simulink model "main_model"  (R2016a)
settings: Solver=VariableStepAuto  StartTime=0.0  StopTime=10.0  RelTol=1e-3
undefined symbols (not defined in the file): K, K_e, K_i
settings Model: Creator=manuel  LastModifiedBy=manuel

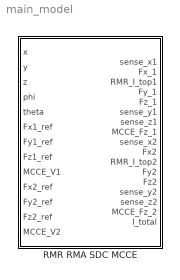
== system main_model ==
  RMR RMA SDC MCCE : Subsystem

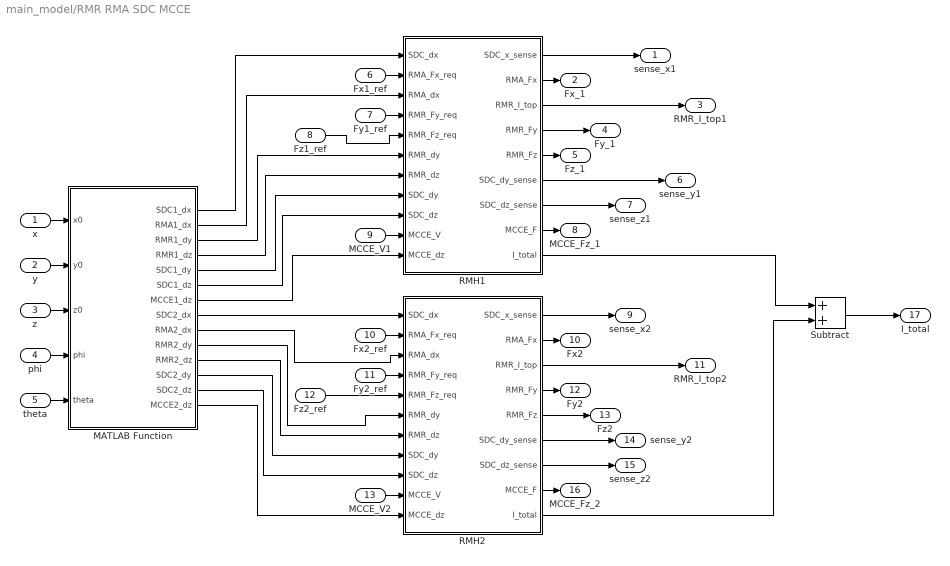
== system main_model/RMR RMA SDC MCCE ==
  x : Inport
  y : Inport  Port=2
  z : Inport  Port=3
  phi : Inport  Port=4
  theta : Inport  Port=5
  Fx1_ref : Inport  Port=6
  Fy1_ref : Inport  Port=7
  Fz1_ref : Inport  Port=8
  MCCE_V1 : Inport  Port=9
  Fx2_ref : Inport  Port=10
  Fy2_ref : Inport  Port=11
  Fz2_ref : Inport  Port=12
  MCCE_V2 : Inport  Port=13
  MATLAB Function : MATLAB Function  TreatAsAtomicUnit=on
  RMH1 : Subsystem
  RMH2 : Subsystem
  Subtract : Sum
  sense_x1 : Outport
  Fx_1 : Outport  Port=2
  RMR_I_top1 : Outport  Port=3
  Fy_1 : Outport  Port=4
  Fz_1 : Outport  Port=5
  sense_y1 : Outport  Port=6
  sense_z1 : Outport  Port=7
  MCCE_Fz_1 : Outport  Port=8
  sense_x2 : Outport  Port=9
  Fx2 : Outport  Port=10
  RMR_I_top2 : Outport  Port=11
  Fy2 : Outport  Port=12
  Fz2 : Outport  Port=13
  sense_y2 : Outport  Port=14
  sense_z2 : Outport  Port=15
  MCCE_Fz_2 : Outport  Port=16
  I_total : Outport  Port=17
  wires:
  MATLAB Function/14(MCCE2_dz) -> RMH2/11(MCCE_dz)
  MATLAB Function/13(SDC2_dz) -> RMH2/9(SDC_dz)
  MATLAB Function/8(SDC2_dx) -> RMH2/1(SDC_dx)
  MATLAB Function/1(SDC1_dx) -> RMH1/1(SDC_dx)
  MATLAB Function/9(RMA2_dx) -> RMH2/3(RMA_dx)
  MATLAB Function/4(RMR1_dz) -> RMH1/7(RMR_dz)
  RMH1/2(RMA_Fx) -> Fx_1/1
  RMH1/7(SDC_dz_sense) -> sense_z1/1
  Fy1_ref/1 -> RMH1/4(RMR_Fy_req)
  Fz1_ref/1 -> RMH1/5(RMR_Fz_req)
  RMH1/4(RMR_Fy) -> Fy_1/1
  RMH1/6(SDC_dy_sense) -> sense_y1/1
  RMH1/1(SDC_x_sense) -> sense_x1/1
  RMH1/3(RMR_I_top) -> RMR_I_top1/1
  RMH1/5(RMR_Fz) -> Fz_1/1
  MCCE_V1/1 -> RMH1/10(MCCE_V)
  Fx1_ref/1 -> RMH1/2(RMA_Fx_req)
  MATLAB Function/7(MCCE1_dz) -> RMH1/11(MCCE_dz)
  MATLAB Function/5(SDC1_dy) -> RMH1/8(SDC_dy)
  MATLAB Function/2(RMA1_dx) -> RMH1/3(RMA_dx)
  RMH2/8(MCCE_F) -> MCCE_Fz_2/1
  y/1 -> MATLAB Function/2(y0)
  x/1 -> MATLAB Function/1(x0)
  RMH2/5(RMR_Fz) -> Fz2/1
  RMH2/3(RMR_I_top) -> RMR_I_top2/1
  z/1 -> MATLAB Function/3(z0)
  phi/1 -> MATLAB Function/4(phi)
  MCCE_V2/1 -> RMH2/10(MCCE_V)
  RMH2/1(SDC_x_sense) -> sense_x2/1
  theta/1 -> MATLAB Function/5(theta)
  RMH1/8(MCCE_F) -> MCCE_Fz_1/1
  Fy2_ref/1 -> RMH2/4(RMR_Fy_req)
  Fz2_ref/1 -> RMH2/5(RMR_Fz_req)
  RMH2/2(RMA_Fx) -> Fx2/1
  Fx2_ref/1 -> RMH2/2(RMA_Fx_req)
  RMH2/4(RMR_Fy) -> Fy2/1
  RMH2/6(SDC_dy_sense) -> sense_y2/1
  RMH2/7(SDC_dz_sense) -> sense_z2/1
  MATLAB Function/10(RMR2_dy) -> RMH2/6(RMR_dy)
  MATLAB Function/3(RMR1_dy) -> RMH1/6(RMR_dy)
  MATLAB Function/12(SDC2_dy) -> RMH2/8(SDC_dy)
  MATLAB Function/6(SDC1_dz) -> RMH1/9(SDC_dz)
  MATLAB Function/11(RMR2_dz) -> RMH2/7(RMR_dz)
  RMH1/9(I_total) -> Subtract/1
  RMH2/9(I_total) -> Subtract/2
  Subtract/1 -> I_total/1

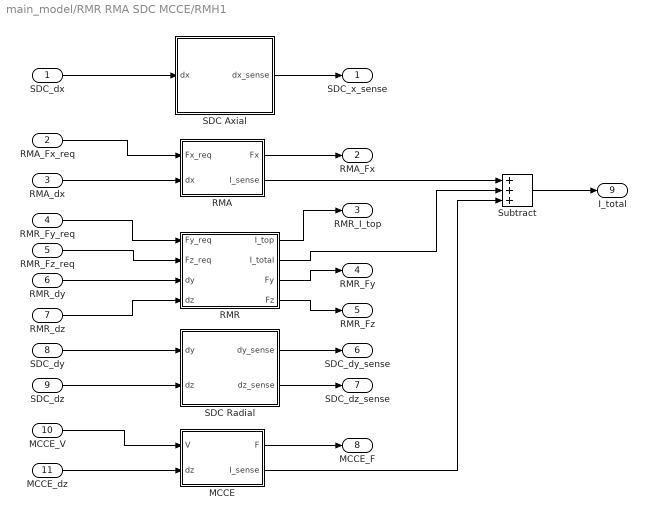
== system main_model/RMR RMA SDC MCCE/RMH1 ==
  SDC_dx : Inport
  RMA_Fx_req : Inport  Port=2
  RMA_dx : Inport  Port=3
  RMR_Fy_req : Inport  Port=4
  RMR_Fz_req : Inport  Port=5
  RMR_dy : Inport  Port=6
  RMR_dz : Inport  Port=7
  SDC_dy : Inport  Port=8
  SDC_dz : Inport  Port=9
  MCCE_V : Inport  Port=10
  MCCE_dz : Inport  Port=11
  MCCE : Subsystem
  RMA : Subsystem
  RMR : Subsystem
  SDC Axial : Subsystem
  SDC Radial : Subsystem
  Subtract : Sum  Inputs=+++
  SDC_x_sense : Outport
  RMA_Fx : Outport  Port=2
  RMR_I_top : Outport  Port=3
  RMR_Fy : Outport  Port=4
  RMR_Fz : Outport  Port=5
  SDC_dy_sense : Outport  Port=6
  SDC_dz_sense : Outport  Port=7
  MCCE_F : Outport  Port=8
  I_total : Outport  Port=9
  wires:
  RMA/1(Fx) -> RMA_Fx/1
  SDC_dy/1 -> SDC Radial/1(dy)
  RMR/4(Fz) -> RMR_Fz/1
  SDC Radial/2(dz_sense) -> SDC_dz_sense/1
  RMA_dx/1 -> RMA/2(dx)
  RMR_dz/1 -> RMR/4(dz)
  MCCE/1(F) -> MCCE_F/1
  RMR_dy/1 -> RMR/3(dy)
  RMR_Fz_req/1 -> RMR/2(Fz_req)
  SDC_dz/1 -> SDC Radial/2(dz)
  SDC Radial/1(dy_sense) -> SDC_dy_sense/1
  MCCE_V/1 -> MCCE/1(V)
  RMR/1(I_top) -> RMR_I_top/1
  MCCE_dz/1 -> MCCE/2(dz)
  RMR_Fy_req/1 -> RMR/1(Fy_req)
  RMR/3(Fy) -> RMR_Fy/1
  RMA_Fx_req/1 -> RMA/1(Fx_req)
  SDC Axial/1(dx_sense) -> SDC_x_sense/1
  SDC_dx/1 -> SDC Axial/1(dx)
  RMR/2(I_total) -> Subtract/2
  RMA/2(I_sense) -> Subtract/1
  MCCE/2(I_sense) -> Subtract/3
  Subtract/1 -> I_total/1

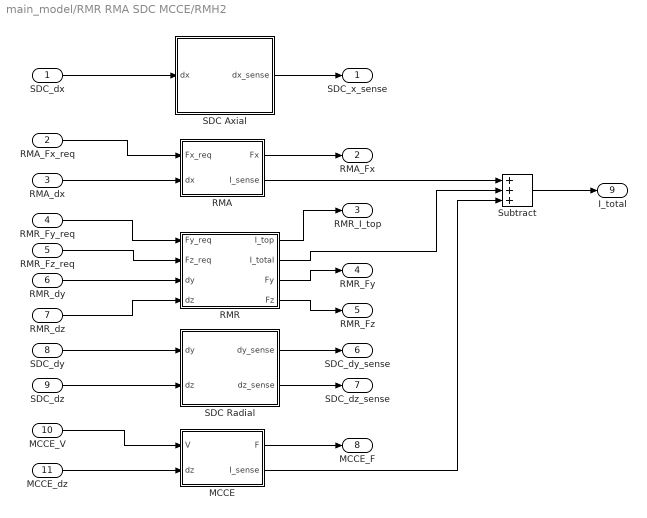
== system main_model/RMR RMA SDC MCCE/RMH2 ==
  SDC_dx : Inport
  RMA_Fx_req : Inport  Port=2
  RMA_dx : Inport  Port=3
  RMR_Fy_req : Inport  Port=4
  RMR_Fz_req : Inport  Port=5
  RMR_dy : Inport  Port=6
  RMR_dz : Inport  Port=7
  SDC_dy : Inport  Port=8
  SDC_dz : Inport  Port=9
  MCCE_V : Inport  Port=10
  MCCE_dz : Inport  Port=11
  MCCE : Subsystem
  RMA : Subsystem
  RMR : Subsystem
  SDC Axial : Subsystem
  SDC Radial : Subsystem
  Subtract : Sum  Inputs=+++
  SDC_x_sense : Outport
  RMA_Fx : Outport  Port=2
  RMR_I_top : Outport  Port=3
  RMR_Fy : Outport  Port=4
  RMR_Fz : Outport  Port=5
  SDC_dy_sense : Outport  Port=6
  SDC_dz_sense : Outport  Port=7
  MCCE_F : Outport  Port=8
  I_total : Outport  Port=9
  wires:
  RMA/1(Fx) -> RMA_Fx/1
  SDC_dy/1 -> SDC Radial/1(dy)
  RMR/4(Fz) -> RMR_Fz/1
  SDC Radial/2(dz_sense) -> SDC_dz_sense/1
  RMA_dx/1 -> RMA/2(dx)
  RMR_dz/1 -> RMR/4(dz)
  MCCE/1(F) -> MCCE_F/1
  RMR_dy/1 -> RMR/3(dy)
  RMR_Fz_req/1 -> RMR/2(Fz_req)
  SDC_dz/1 -> SDC Radial/2(dz)
  SDC Radial/1(dy_sense) -> SDC_dy_sense/1
  MCCE_V/1 -> MCCE/1(V)
  RMR/1(I_top) -> RMR_I_top/1
  MCCE_dz/1 -> MCCE/2(dz)
  RMR_Fy_req/1 -> RMR/1(Fy_req)
  RMR/3(Fy) -> RMR_Fy/1
  RMA_Fx_req/1 -> RMA/1(Fx_req)
  SDC Axial/1(dx_sense) -> SDC_x_sense/1
  SDC_dx/1 -> SDC Axial/1(dx)
  RMR/2(I_total) -> Subtract/2
  RMA/2(I_sense) -> Subtract/1
  MCCE/2(I_sense) -> Subtract/3
  Subtract/1 -> I_total/1

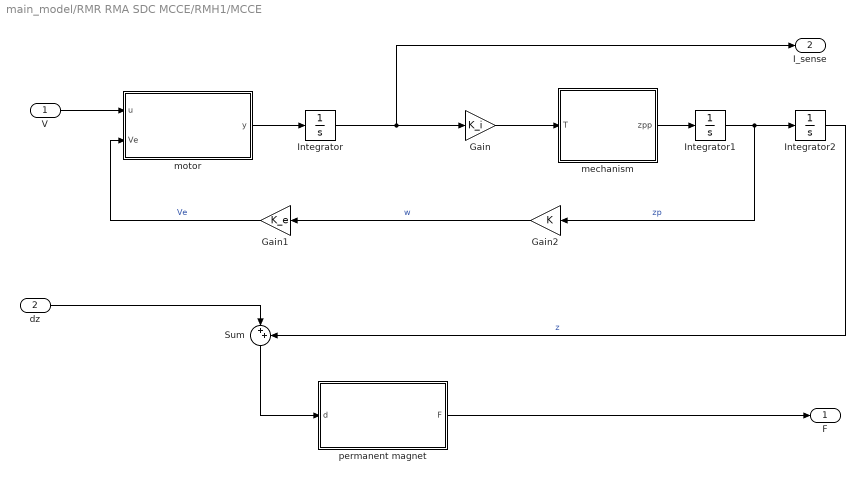
== system main_model/RMR RMA SDC MCCE/RMH1/MCCE ==
  V : Inport
  dz : Inport  Port=2
  Gain : Gain  Gain=K_i
  Gain1 : Gain  Gain=K_e
  Gain2 : Gain  Gain=K
  Integrator : Integrator
  Integrator1 : Integrator
  Integrator2 : Integrator
  Sum : Sum  Inputs=|++
  mechanism : MATLAB Function  TreatAsAtomicUnit=on
  motor : MATLAB Function  TreatAsAtomicUnit=on
  permanent magnet : MATLAB Function  TreatAsAtomicUnit=on
  F : Outport
  I_sense : Outport  Port=2
  wires:
  V/1 -> motor/1(u)
  dz/1 -> Sum/1
  Sum/1 -> permanent magnet/1(d)
  motor/1(y) -> Integrator/1
  Integrator/1 -> I_sense/1, Gain/1
  Gain/1 -> mechanism/1(T)
  mechanism/1(zpp) -> Integrator1/1
  Gain1/1 -> motor/2(Ve)  "Ve"
  Gain2/1 -> Gain1/1  "w"
  Integrator2/1 -> Sum/2  "z"
  Integrator1/1 -> Gain2/1, Integrator2/1  "zp"
  permanent magnet/1(F) -> F/1

== system main_model/RMR RMA SDC MCCE/RMH1/RMA ==
  Fx_req : Inport
  dx : Inport  Port=2
  FB Linearized EIA1 : Subsystem
  Force Selector : MATLAB Function  TreatAsAtomicUnit=on
  Fx : Outport
  I_sense : Outport  Port=2
  wires:
  Fx_req/1 -> Force Selector/1(Fx)
  Force Selector/1(F1) -> FB Linearized EIA1/1(F_ref)
  dx/1 -> FB Linearized EIA1/2(d)
  FB Linearized EIA1/2(F) -> Fx/1
  FB Linearized EIA1/1(I_sense) -> I_sense/1

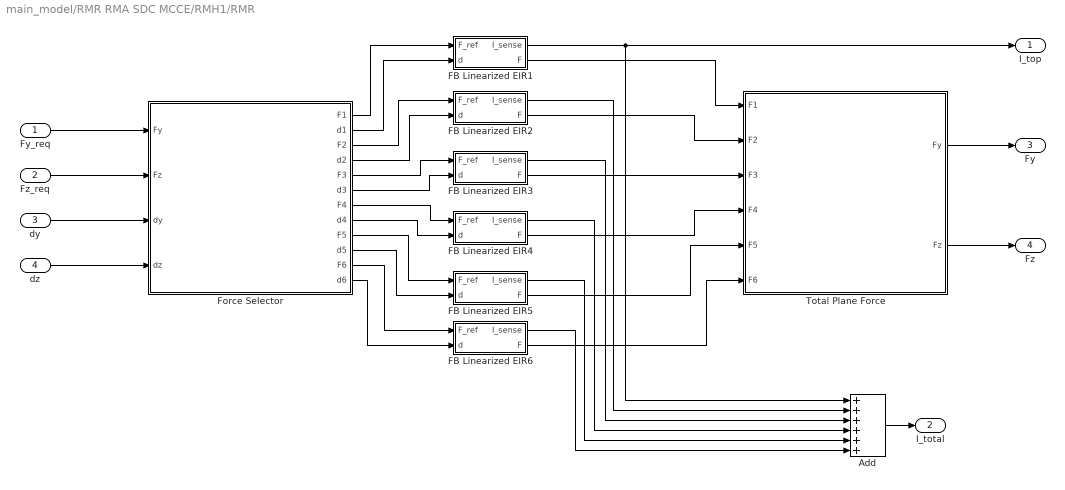
== system main_model/RMR RMA SDC MCCE/RMH1/RMR ==
  Fy_req : Inport
  Fz_req : Inport  Port=2
  dy : Inport  Port=3
  dz : Inport  Port=4
  Add : Sum  Inputs=++++++
  FB Linearized EIR1 : Subsystem
  FB Linearized EIR2 : Subsystem
  FB Linearized EIR3 : Subsystem
  FB Linearized EIR4 : Subsystem
  FB Linearized EIR5 : Subsystem
  FB Linearized EIR6 : Subsystem
  Force Selector : MATLAB Function  TreatAsAtomicUnit=on
  Total Plane Force : MATLAB Function  TreatAsAtomicUnit=on
  I_top : Outport
  I_total : Outport  Port=2
  Fy : Outport  Port=3
  Fz : Outport  Port=4
  wires:
  dy/1 -> Force Selector/3(dy)
  Total Plane Force/2(Fz) -> Fz/1
  Fy_req/1 -> Force Selector/1(Fy)
  Force Selector/7(F4) -> FB Linearized EIR4/1(F_ref)
  dz/1 -> Force Selector/4(dz)
  Force Selector/1(F1) -> FB Linearized EIR1/1(F_ref)
  Force Selector/4(d2) -> FB Linearized EIR2/2(d)
  FB Linearized EIR4/2(F) -> Total Plane Force/4(F4)
  FB Linearized EIR6/2(F) -> Total Plane Force/6(F6)
  Fz_req/1 -> Force Selector/2(Fz)
  Total Plane Force/1(Fy) -> Fy/1
  Force Selector/3(F2) -> FB Linearized EIR2/1(F_ref)
  Force Selector/2(d1) -> FB Linearized EIR1/2(d)
  Force Selector/11(F6) -> FB Linearized EIR6/1(F_ref)
  Force Selector/9(F5) -> FB Linearized EIR5/1(F_ref)
  Force Selector/8(d4) -> FB Linearized EIR4/2(d)
  FB Linearized EIR3/2(F) -> Total Plane Force/3(F3)
  Force Selector/10(d5) -> FB Linearized EIR5/2(d)
  FB Linearized EIR1/1(I_sense) -> I_top/1, Add/1
  FB Linearized EIR1/2(F) -> Total Plane Force/1(F1)
  Force Selector/5(F3) -> FB Linearized EIR3/1(F_ref)
  Force Selector/6(d3) -> FB Linearized EIR3/2(d)
  FB Linearized EIR2/2(F) -> Total Plane Force/2(F2)
  Force Selector/12(d6) -> FB Linearized EIR6/2(d)
  FB Linearized EIR5/2(F) -> Total Plane Force/5(F5)
  Add/1 -> I_total/1
  FB Linearized EIR2/1(I_sense) -> Add/2
  FB Linearized EIR3/1(I_sense) -> Add/3
  FB Linearized EIR4/1(I_sense) -> Add/4
  FB Linearized EIR5/1(I_sense) -> Add/5
  FB Linearized EIR6/1(I_sense) -> Add/6

== system main_model/RMR RMA SDC MCCE/RMH1/SDC Axial ==
  dx : Inport
  SDC Axial 1 : MATLAB Function  TreatAsAtomicUnit=on
  dx_sense : Outport
  wires:
  dx/1 -> SDC Axial 1/1(d_real)
  SDC Axial 1/1(d_sense) -> dx_sense/1

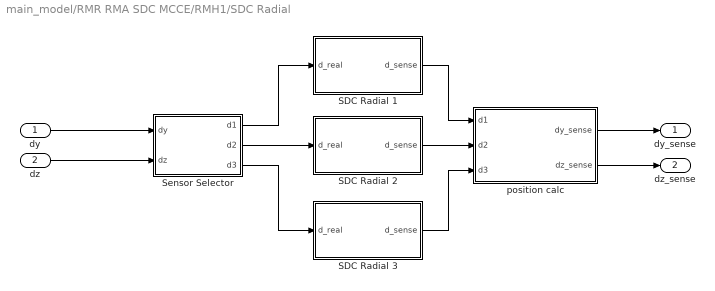
== system main_model/RMR RMA SDC MCCE/RMH1/SDC Radial ==
  dy : Inport
  dz : Inport  Port=2
  SDC Radial 1 : MATLAB Function  TreatAsAtomicUnit=on
  SDC Radial 2 : MATLAB Function  TreatAsAtomicUnit=on
  SDC Radial 3 : MATLAB Function  TreatAsAtomicUnit=on
  Sensor Selector : MATLAB Function  TreatAsAtomicUnit=on
  position calc : MATLAB Function  TreatAsAtomicUnit=on
  dy_sense : Outport
  dz_sense : Outport  Port=2
  wires:
  dy/1 -> Sensor Selector/1(dy)
  dz/1 -> Sensor Selector/2(dz)
  Sensor Selector/1(d1) -> SDC Radial 1/1(d_real)
  Sensor Selector/2(d2) -> SDC Radial 2/1(d_real)
  Sensor Selector/3(d3) -> SDC Radial 3/1(d_real)
  SDC Radial 2/1(d_sense) -> position calc/2(d2)
  SDC Radial 1/1(d_sense) -> position calc/1(d1)
  SDC Radial 3/1(d_sense) -> position calc/3(d3)
  position calc/1(dy_sense) -> dy_sense/1
  position calc/2(dz_sense) -> dz_sense/1

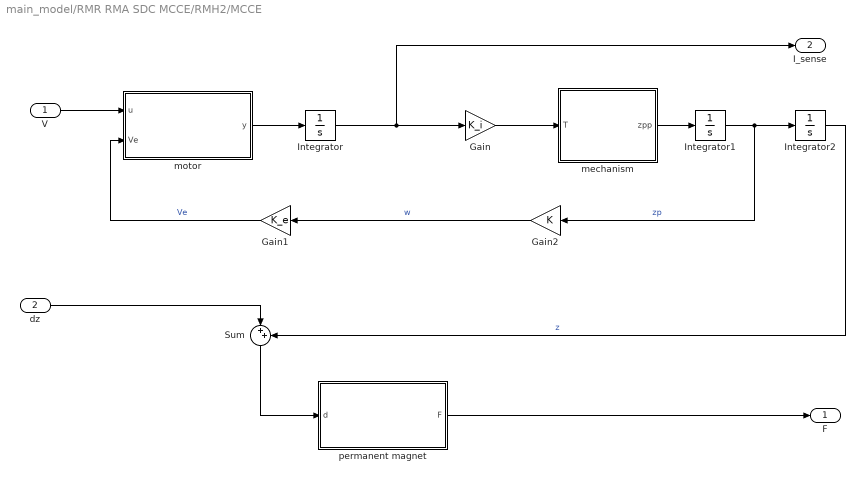
== system main_model/RMR RMA SDC MCCE/RMH2/MCCE ==
  V : Inport
  dz : Inport  Port=2
  Gain : Gain  Gain=K_i
  Gain1 : Gain  Gain=K_e
  Gain2 : Gain  Gain=K
  Integrator : Integrator
  Integrator1 : Integrator
  Integrator2 : Integrator
  Sum : Sum  Inputs=|++
  mechanism : MATLAB Function  TreatAsAtomicUnit=on
  motor : MATLAB Function  TreatAsAtomicUnit=on
  permanent magnet : MATLAB Function  TreatAsAtomicUnit=on
  F : Outport
  I_sense : Outport  Port=2
  wires:
  V/1 -> motor/1(u)
  dz/1 -> Sum/1
  Sum/1 -> permanent magnet/1(d)
  motor/1(y) -> Integrator/1
  Integrator/1 -> I_sense/1, Gain/1
  Gain/1 -> mechanism/1(T)
  mechanism/1(zpp) -> Integrator1/1
  Gain1/1 -> motor/2(Ve)  "Ve"
  Gain2/1 -> Gain1/1  "w"
  Integrator2/1 -> Sum/2  "z"
  Integrator1/1 -> Gain2/1, Integrator2/1  "zp"
  permanent magnet/1(F) -> F/1

== system main_model/RMR RMA SDC MCCE/RMH2/RMA ==
  Fx_req : Inport
  dx : Inport  Port=2
  FB Linearized EIA1 : Subsystem
  Force Selector : MATLAB Function  TreatAsAtomicUnit=on
  Fx : Outport
  I_sense : Outport  Port=2
  wires:
  Fx_req/1 -> Force Selector/1(Fx)
  Force Selector/1(F1) -> FB Linearized EIA1/1(F_ref)
  dx/1 -> FB Linearized EIA1/2(d)
  FB Linearized EIA1/2(F) -> Fx/1
  FB Linearized EIA1/1(I_sense) -> I_sense/1

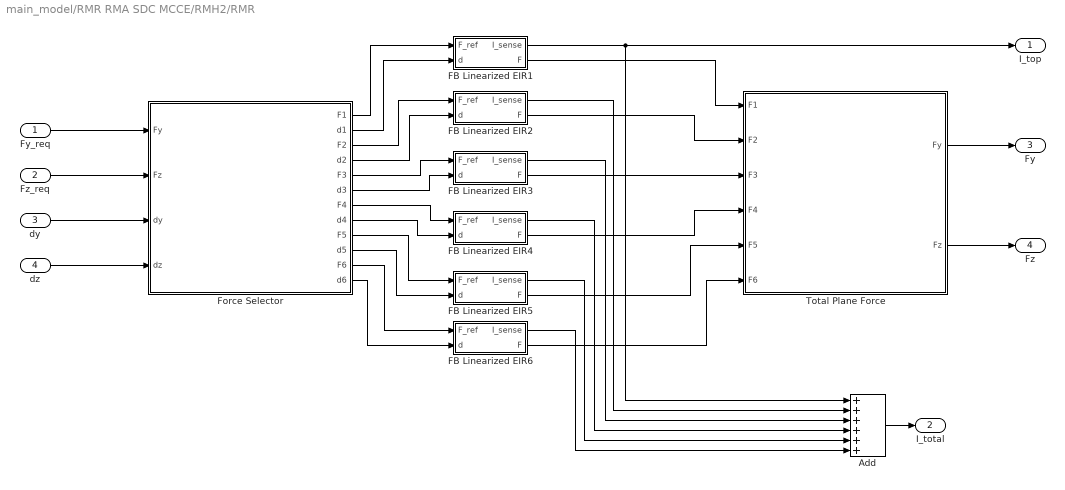
== system main_model/RMR RMA SDC MCCE/RMH2/RMR ==
  Fy_req : Inport
  Fz_req : Inport  Port=2
  dy : Inport  Port=3
  dz : Inport  Port=4
  Add : Sum  Inputs=++++++
  FB Linearized EIR1 : Subsystem
  FB Linearized EIR2 : Subsystem
  FB Linearized EIR3 : Subsystem
  FB Linearized EIR4 : Subsystem
  FB Linearized EIR5 : Subsystem
  FB Linearized EIR6 : Subsystem
  Force Selector : MATLAB Function  TreatAsAtomicUnit=on
  Total Plane Force : MATLAB Function  TreatAsAtomicUnit=on
  I_top : Outport
  I_total : Outport  Port=2
  Fy : Outport  Port=3
  Fz : Outport  Port=4
  wires:
  dy/1 -> Force Selector/3(dy)
  Total Plane Force/2(Fz) -> Fz/1
  Fy_req/1 -> Force Selector/1(Fy)
  Force Selector/7(F4) -> FB Linearized EIR4/1(F_ref)
  dz/1 -> Force Selector/4(dz)
  Force Selector/1(F1) -> FB Linearized EIR1/1(F_ref)
  Force Selector/4(d2) -> FB Linearized EIR2/2(d)
  FB Linearized EIR4/2(F) -> Total Plane Force/4(F4)
  FB Linearized EIR6/2(F) -> Total Plane Force/6(F6)
  Fz_req/1 -> Force Selector/2(Fz)
  Total Plane Force/1(Fy) -> Fy/1
  Force Selector/3(F2) -> FB Linearized EIR2/1(F_ref)
  Force Selector/2(d1) -> FB Linearized EIR1/2(d)
  Force Selector/11(F6) -> FB Linearized EIR6/1(F_ref)
  Force Selector/9(F5) -> FB Linearized EIR5/1(F_ref)
  Force Selector/8(d4) -> FB Linearized EIR4/2(d)
  FB Linearized EIR3/2(F) -> Total Plane Force/3(F3)
  Force Selector/10(d5) -> FB Linearized EIR5/2(d)
  FB Linearized EIR1/1(I_sense) -> I_top/1, Add/1
  FB Linearized EIR1/2(F) -> Total Plane Force/1(F1)
  Force Selector/5(F3) -> FB Linearized EIR3/1(F_ref)
  Force Selector/6(d3) -> FB Linearized EIR3/2(d)
  FB Linearized EIR2/2(F) -> Total Plane Force/2(F2)
  Force Selector/12(d6) -> FB Linearized EIR6/2(d)
  FB Linearized EIR5/2(F) -> Total Plane Force/5(F5)
  Add/1 -> I_total/1
  FB Linearized EIR2/1(I_sense) -> Add/2
  FB Linearized EIR3/1(I_sense) -> Add/3
  FB Linearized EIR4/1(I_sense) -> Add/4
  FB Linearized EIR5/1(I_sense) -> Add/5
  FB Linearized EIR6/1(I_sense) -> Add/6

== system main_model/RMR RMA SDC MCCE/RMH2/SDC Axial ==
  dx : Inport
  SDC Axial 1 : MATLAB Function  TreatAsAtomicUnit=on
  dx_sense : Outport
  wires:
  dx/1 -> SDC Axial 1/1(d_real)
  SDC Axial 1/1(d_sense) -> dx_sense/1

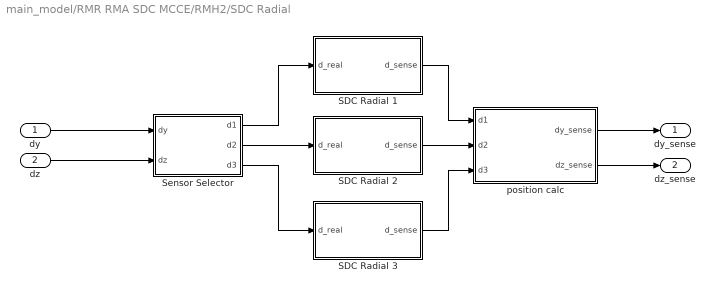
== system main_model/RMR RMA SDC MCCE/RMH2/SDC Radial ==
  dy : Inport
  dz : Inport  Port=2
  SDC Radial 1 : MATLAB Function  TreatAsAtomicUnit=on
  SDC Radial 2 : MATLAB Function  TreatAsAtomicUnit=on
  SDC Radial 3 : MATLAB Function  TreatAsAtomicUnit=on
  Sensor Selector : MATLAB Function  TreatAsAtomicUnit=on
  position calc : MATLAB Function  TreatAsAtomicUnit=on
  dy_sense : Outport
  dz_sense : Outport  Port=2
  wires:
  dy/1 -> Sensor Selector/1(dy)
  dz/1 -> Sensor Selector/2(dz)
  Sensor Selector/1(d1) -> SDC Radial 1/1(d_real)
  Sensor Selector/2(d2) -> SDC Radial 2/1(d_real)
  Sensor Selector/3(d3) -> SDC Radial 3/1(d_real)
  SDC Radial 2/1(d_sense) -> position calc/2(d2)
  SDC Radial 1/1(d_sense) -> position calc/1(d1)
  SDC Radial 3/1(d_sense) -> position calc/3(d3)
  position calc/1(dy_sense) -> dy_sense/1
  position calc/2(dz_sense) -> dz_sense/1

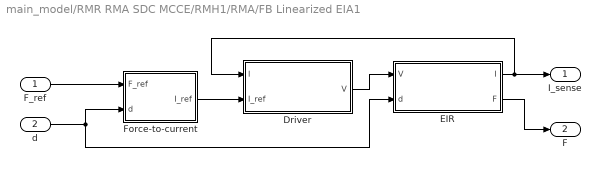
== system main_model/RMR RMA SDC MCCE/RMH1/RMA/FB Linearized EIA1 ==
  F_ref : Inport
  d : Inport  Port=2
  Driver : Subsystem
  EIR : Subsystem
  Force-to-current : MATLAB Function  TreatAsAtomicUnit=on
  I_sense : Outport
  F : Outport  Port=2
  wires:
  Driver/1(V) -> EIR/1(V)
  d/1 -> EIR/2(d), Force-to-current/2(d)
  F_ref/1 -> Force-to-current/1(F_ref)
  Force-to-current/1(I_ref) -> Driver/2(I_ref)
  EIR/2(F) -> F/1
  EIR/1(I) -> Driver/1("I "), I_sense/1

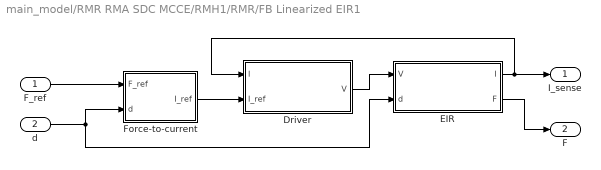
== system main_model/RMR RMA SDC MCCE/RMH1/RMR/FB Linearized EIR1 ==
  F_ref : Inport
  d : Inport  Port=2
  Driver : Subsystem
  EIR : Subsystem
  Force-to-current : MATLAB Function  TreatAsAtomicUnit=on
  I_sense : Outport
  F : Outport  Port=2
  wires:
  Driver/1(V) -> EIR/1(V)
  d/1 -> EIR/2(d), Force-to-current/2(d)
  F_ref/1 -> Force-to-current/1(F_ref)
  Force-to-current/1(I_ref) -> Driver/2(I_ref)
  EIR/2(F) -> F/1
  EIR/1(I) -> Driver/1("I "), I_sense/1

== system main_model/RMR RMA SDC MCCE/RMH1/RMR/FB Linearized EIR2 ==
  F_ref : Inport
  d : Inport  Port=2
  Driver : Subsystem
  EIR : Subsystem
  Force-to-current : MATLAB Function  TreatAsAtomicUnit=on
  I_sense : Outport
  F : Outport  Port=2
  wires:
  Driver/1(V) -> EIR/1(V)
  d/1 -> EIR/2(d), Force-to-current/2(d)
  F_ref/1 -> Force-to-current/1(F_ref)
  Force-to-current/1(I_ref) -> Driver/2(I_ref)
  EIR/2(F) -> F/1
  EIR/1(I) -> Driver/1("I "), I_sense/1

== system main_model/RMR RMA SDC MCCE/RMH1/RMR/FB Linearized EIR3 ==
  F_ref : Inport
  d : Inport  Port=2
  Driver : Subsystem
  EIR : Subsystem
  Force-to-current : MATLAB Function  TreatAsAtomicUnit=on
  I_sense : Outport
  F : Outport  Port=2
  wires:
  Driver/1(V) -> EIR/1(V)
  d/1 -> EIR/2(d), Force-to-current/2(d)
  F_ref/1 -> Force-to-current/1(F_ref)
  Force-to-current/1(I_ref) -> Driver/2(I_ref)
  EIR/2(F) -> F/1
  EIR/1(I) -> Driver/1("I "), I_sense/1

== system main_model/RMR RMA SDC MCCE/RMH1/RMR/FB Linearized EIR4 ==
  F_ref : Inport
  d : Inport  Port=2
  Driver : Subsystem
  EIR : Subsystem
  Force-to-current : MATLAB Function  TreatAsAtomicUnit=on
  I_sense : Outport
  F : Outport  Port=2
  wires:
  Driver/1(V) -> EIR/1(V)
  d/1 -> EIR/2(d), Force-to-current/2(d)
  F_ref/1 -> Force-to-current/1(F_ref)
  Force-to-current/1(I_ref) -> Driver/2(I_ref)
  EIR/2(F) -> F/1
  EIR/1(I) -> Driver/1("I "), I_sense/1

== system main_model/RMR RMA SDC MCCE/RMH1/RMR/FB Linearized EIR5 ==
  F_ref : Inport
  d : Inport  Port=2
  Driver : Subsystem
  EIR : Subsystem
  Force-to-current : MATLAB Function  TreatAsAtomicUnit=on
  I_sense : Outport
  F : Outport  Port=2
  wires:
  Driver/1(V) -> EIR/1(V)
  d/1 -> EIR/2(d), Force-to-current/2(d)
  F_ref/1 -> Force-to-current/1(F_ref)
  Force-to-current/1(I_ref) -> Driver/2(I_ref)
  EIR/2(F) -> F/1
  EIR/1(I) -> Driver/1("I "), I_sense/1

== system main_model/RMR RMA SDC MCCE/RMH1/RMR/FB Linearized EIR6 ==
  F_ref : Inport
  d : Inport  Port=2
  Driver : Subsystem
  EIR : Subsystem
  Force-to-current : MATLAB Function  TreatAsAtomicUnit=on
  I_sense : Outport
  F : Outport  Port=2
  wires:
  Driver/1(V) -> EIR/1(V)
  d/1 -> EIR/2(d), Force-to-current/2(d)
  F_ref/1 -> Force-to-current/1(F_ref)
  Force-to-current/1(I_ref) -> Driver/2(I_ref)
  EIR/2(F) -> F/1
  EIR/1(I) -> Driver/1("I "), I_sense/1

== system main_model/RMR RMA SDC MCCE/RMH2/RMA/FB Linearized EIA1 ==
  F_ref : Inport
  d : Inport  Port=2
  Driver : Subsystem
  EIR : Subsystem
  Force-to-current : MATLAB Function  TreatAsAtomicUnit=on
  I_sense : Outport
  F : Outport  Port=2
  wires:
  Driver/1(V) -> EIR/1(V)
  d/1 -> EIR/2(d), Force-to-current/2(d)
  F_ref/1 -> Force-to-current/1(F_ref)
  Force-to-current/1(I_ref) -> Driver/2(I_ref)
  EIR/2(F) -> F/1
  EIR/1(I) -> Driver/1("I "), I_sense/1

== system main_model/RMR RMA SDC MCCE/RMH2/RMR/FB Linearized EIR1 ==
  F_ref : Inport
  d : Inport  Port=2
  Driver : Subsystem
  EIR : Subsystem
  Force-to-current : MATLAB Function  TreatAsAtomicUnit=on
  I_sense : Outport
  F : Outport  Port=2
  wires:
  Driver/1(V) -> EIR/1(V)
  d/1 -> EIR/2(d), Force-to-current/2(d)
  F_ref/1 -> Force-to-current/1(F_ref)
  Force-to-current/1(I_ref) -> Driver/2(I_ref)
  EIR/2(F) -> F/1
  EIR/1(I) -> Driver/1("I "), I_sense/1

== system main_model/RMR RMA SDC MCCE/RMH2/RMR/FB Linearized EIR2 ==
  F_ref : Inport
  d : Inport  Port=2
  Driver : Subsystem
  EIR : Subsystem
  Force-to-current : MATLAB Function  TreatAsAtomicUnit=on
  I_sense : Outport
  F : Outport  Port=2
  wires:
  Driver/1(V) -> EIR/1(V)
  d/1 -> EIR/2(d), Force-to-current/2(d)
  F_ref/1 -> Force-to-current/1(F_ref)
  Force-to-current/1(I_ref) -> Driver/2(I_ref)
  EIR/2(F) -> F/1
  EIR/1(I) -> Driver/1("I "), I_sense/1

== system main_model/RMR RMA SDC MCCE/RMH2/RMR/FB Linearized EIR3 ==
  F_ref : Inport
  d : Inport  Port=2
  Driver : Subsystem
  EIR : Subsystem
  Force-to-current : MATLAB Function  TreatAsAtomicUnit=on
  I_sense : Outport
  F : Outport  Port=2
  wires:
  Driver/1(V) -> EIR/1(V)
  d/1 -> EIR/2(d), Force-to-current/2(d)
  F_ref/1 -> Force-to-current/1(F_ref)
  Force-to-current/1(I_ref) -> Driver/2(I_ref)
  EIR/2(F) -> F/1
  EIR/1(I) -> Driver/1("I "), I_sense/1

== system main_model/RMR RMA SDC MCCE/RMH2/RMR/FB Linearized EIR4 ==
  F_ref : Inport
  d : Inport  Port=2
  Driver : Subsystem
  EIR : Subsystem
  Force-to-current : MATLAB Function  TreatAsAtomicUnit=on
  I_sense : Outport
  F : Outport  Port=2
  wires:
  Driver/1(V) -> EIR/1(V)
  d/1 -> EIR/2(d), Force-to-current/2(d)
  F_ref/1 -> Force-to-current/1(F_ref)
  Force-to-current/1(I_ref) -> Driver/2(I_ref)
  EIR/2(F) -> F/1
  EIR/1(I) -> Driver/1("I "), I_sense/1

== system main_model/RMR RMA SDC MCCE/RMH2/RMR/FB Linearized EIR5 ==
  F_ref : Inport
  d : Inport  Port=2
  Driver : Subsystem
  EIR : Subsystem
  Force-to-current : MATLAB Function  TreatAsAtomicUnit=on
  I_sense : Outport
  F : Outport  Port=2
  wires:
  Driver/1(V) -> EIR/1(V)
  d/1 -> EIR/2(d), Force-to-current/2(d)
  F_ref/1 -> Force-to-current/1(F_ref)
  Force-to-current/1(I_ref) -> Driver/2(I_ref)
  EIR/2(F) -> F/1
  EIR/1(I) -> Driver/1("I "), I_sense/1

== system main_model/RMR RMA SDC MCCE/RMH2/RMR/FB Linearized EIR6 ==
  F_ref : Inport
  d : Inport  Port=2
  Driver : Subsystem
  EIR : Subsystem
  Force-to-current : MATLAB Function  TreatAsAtomicUnit=on
  I_sense : Outport
  F : Outport  Port=2
  wires:
  Driver/1(V) -> EIR/1(V)
  d/1 -> EIR/2(d), Force-to-current/2(d)
  F_ref/1 -> Force-to-current/1(F_ref)
  Force-to-current/1(I_ref) -> Driver/2(I_ref)
  EIR/2(F) -> F/1
  EIR/1(I) -> Driver/1("I "), I_sense/1

== system main_model/RMR RMA SDC MCCE/RMH1/RMA/FB Linearized EIA1/Driver ==
  "I " : Inport
  I_ref : Inport  Port=2
  Gain : Gain  Gain=K
  Saturation : Saturate
  Sum : Sum  Inputs=|+-
  V : Outport
  wires:
  Saturation/1 -> V/1
  Sum/1 -> Gain/1
  Gain/1 -> Saturation/1
  "I "/1 -> Sum/2
  I_ref/1 -> Sum/1

== system main_model/RMR RMA SDC MCCE/RMH1/RMA/FB Linearized EIA1/EIR ==
  V : Inport
  d : Inport  Port=2
  Electromagnet : MATLAB Function  TreatAsAtomicUnit=on
  Integrator : Integrator
  I : Outport
  F : Outport  Port=2
  wires:
  Integrator/1 -> Electromagnet/1(I), I/1
  Electromagnet/1(dI_dt) -> Integrator/1
  Electromagnet/2(F) -> F/1
  V/1 -> Electromagnet/2(V)
  d/1 -> Electromagnet/3(d)

== system main_model/RMR RMA SDC MCCE/RMH1/RMR/FB Linearized EIR1/Driver ==
  "I " : Inport
  I_ref : Inport  Port=2
  Gain : Gain  Gain=K
  Saturation : Saturate
  Sum : Sum  Inputs=|+-
  V : Outport
  wires:
  Saturation/1 -> V/1
  Sum/1 -> Gain/1
  Gain/1 -> Saturation/1
  "I "/1 -> Sum/2
  I_ref/1 -> Sum/1

== system main_model/RMR RMA SDC MCCE/RMH1/RMR/FB Linearized EIR1/EIR ==
  V : Inport
  d : Inport  Port=2
  Electromagnet : MATLAB Function  TreatAsAtomicUnit=on
  Integrator : Integrator
  I : Outport
  F : Outport  Port=2
  wires:
  Integrator/1 -> Electromagnet/1(I), I/1
  Electromagnet/1(dI_dt) -> Integrator/1
  Electromagnet/2(F) -> F/1
  V/1 -> Electromagnet/2(V)
  d/1 -> Electromagnet/3(d)

== system main_model/RMR RMA SDC MCCE/RMH1/RMR/FB Linearized EIR2/Driver ==
  "I " : Inport
  I_ref : Inport  Port=2
  Gain : Gain  Gain=K
  Saturation : Saturate
  Sum : Sum  Inputs=|+-
  V : Outport
  wires:
  Saturation/1 -> V/1
  Sum/1 -> Gain/1
  Gain/1 -> Saturation/1
  "I "/1 -> Sum/2
  I_ref/1 -> Sum/1

== system main_model/RMR RMA SDC MCCE/RMH1/RMR/FB Linearized EIR2/EIR ==
  V : Inport
  d : Inport  Port=2
  Electromagnet : MATLAB Function  TreatAsAtomicUnit=on
  Integrator : Integrator
  I : Outport
  F : Outport  Port=2
  wires:
  Integrator/1 -> Electromagnet/1(I), I/1
  Electromagnet/1(dI_dt) -> Integrator/1
  Electromagnet/2(F) -> F/1
  V/1 -> Electromagnet/2(V)
  d/1 -> Electromagnet/3(d)

== system main_model/RMR RMA SDC MCCE/RMH1/RMR/FB Linearized EIR3/Driver ==
  "I " : Inport
  I_ref : Inport  Port=2
  Gain : Gain  Gain=K
  Saturation : Saturate
  Sum : Sum  Inputs=|+-
  V : Outport
  wires:
  Saturation/1 -> V/1
  Sum/1 -> Gain/1
  Gain/1 -> Saturation/1
  "I "/1 -> Sum/2
  I_ref/1 -> Sum/1

== system main_model/RMR RMA SDC MCCE/RMH1/RMR/FB Linearized EIR3/EIR ==
  V : Inport
  d : Inport  Port=2
  Electromagnet : MATLAB Function  TreatAsAtomicUnit=on
  Integrator : Integrator
  I : Outport
  F : Outport  Port=2
  wires:
  Integrator/1 -> Electromagnet/1(I), I/1
  Electromagnet/1(dI_dt) -> Integrator/1
  Electromagnet/2(F) -> F/1
  V/1 -> Electromagnet/2(V)
  d/1 -> Electromagnet/3(d)

== system main_model/RMR RMA SDC MCCE/RMH1/RMR/FB Linearized EIR4/Driver ==
  "I " : Inport
  I_ref : Inport  Port=2
  Gain : Gain  Gain=K
  Saturation : Saturate
  Sum : Sum  Inputs=|+-
  V : Outport
  wires:
  Saturation/1 -> V/1
  Sum/1 -> Gain/1
  Gain/1 -> Saturation/1
  "I "/1 -> Sum/2
  I_ref/1 -> Sum/1

== system main_model/RMR RMA SDC MCCE/RMH1/RMR/FB Linearized EIR4/EIR ==
  V : Inport
  d : Inport  Port=2
  Electromagnet : MATLAB Function  TreatAsAtomicUnit=on
  Integrator : Integrator
  I : Outport
  F : Outport  Port=2
  wires:
  Integrator/1 -> Electromagnet/1(I), I/1
  Electromagnet/1(dI_dt) -> Integrator/1
  Electromagnet/2(F) -> F/1
  V/1 -> Electromagnet/2(V)
  d/1 -> Electromagnet/3(d)

== system main_model/RMR RMA SDC MCCE/RMH1/RMR/FB Linearized EIR5/Driver ==
  "I " : Inport
  I_ref : Inport  Port=2
  Gain : Gain  Gain=K
  Saturation : Saturate
  Sum : Sum  Inputs=|+-
  V : Outport
  wires:
  Saturation/1 -> V/1
  Sum/1 -> Gain/1
  Gain/1 -> Saturation/1
  "I "/1 -> Sum/2
  I_ref/1 -> Sum/1

== system main_model/RMR RMA SDC MCCE/RMH1/RMR/FB Linearized EIR5/EIR ==
  V : Inport
  d : Inport  Port=2
  Electromagnet : MATLAB Function  TreatAsAtomicUnit=on
  Integrator : Integrator
  I : Outport
  F : Outport  Port=2
  wires:
  Integrator/1 -> Electromagnet/1(I), I/1
  Electromagnet/1(dI_dt) -> Integrator/1
  Electromagnet/2(F) -> F/1
  V/1 -> Electromagnet/2(V)
  d/1 -> Electromagnet/3(d)

== system main_model/RMR RMA SDC MCCE/RMH1/RMR/FB Linearized EIR6/Driver ==
  "I " : Inport
  I_ref : Inport  Port=2
  Gain : Gain  Gain=K
  Saturation : Saturate
  Sum : Sum  Inputs=|+-
  V : Outport
  wires:
  Saturation/1 -> V/1
  Sum/1 -> Gain/1
  Gain/1 -> Saturation/1
  "I "/1 -> Sum/2
  I_ref/1 -> Sum/1

== system main_model/RMR RMA SDC MCCE/RMH1/RMR/FB Linearized EIR6/EIR ==
  V : Inport
  d : Inport  Port=2
  Electromagnet : MATLAB Function  TreatAsAtomicUnit=on
  Integrator : Integrator
  I : Outport
  F : Outport  Port=2
  wires:
  Integrator/1 -> Electromagnet/1(I), I/1
  Electromagnet/1(dI_dt) -> Integrator/1
  Electromagnet/2(F) -> F/1
  V/1 -> Electromagnet/2(V)
  d/1 -> Electromagnet/3(d)

== system main_model/RMR RMA SDC MCCE/RMH2/RMA/FB Linearized EIA1/Driver ==
  "I " : Inport
  I_ref : Inport  Port=2
  Gain : Gain  Gain=K
  Saturation : Saturate
  Sum : Sum  Inputs=|+-
  V : Outport
  wires:
  Saturation/1 -> V/1
  Sum/1 -> Gain/1
  Gain/1 -> Saturation/1
  "I "/1 -> Sum/2
  I_ref/1 -> Sum/1

== system main_model/RMR RMA SDC MCCE/RMH2/RMA/FB Linearized EIA1/EIR ==
  V : Inport
  d : Inport  Port=2
  Electromagnet : MATLAB Function  TreatAsAtomicUnit=on
  Integrator : Integrator
  I : Outport
  F : Outport  Port=2
  wires:
  Integrator/1 -> Electromagnet/1(I), I/1
  Electromagnet/1(dI_dt) -> Integrator/1
  Electromagnet/2(F) -> F/1
  V/1 -> Electromagnet/2(V)
  d/1 -> Electromagnet/3(d)

== system main_model/RMR RMA SDC MCCE/RMH2/RMR/FB Linearized EIR1/Driver ==
  "I " : Inport
  I_ref : Inport  Port=2
  Gain : Gain  Gain=K
  Saturation : Saturate
  Sum : Sum  Inputs=|+-
  V : Outport
  wires:
  Saturation/1 -> V/1
  Sum/1 -> Gain/1
  Gain/1 -> Saturation/1
  "I "/1 -> Sum/2
  I_ref/1 -> Sum/1

== system main_model/RMR RMA SDC MCCE/RMH2/RMR/FB Linearized EIR1/EIR ==
  V : Inport
  d : Inport  Port=2
  Electromagnet : MATLAB Function  TreatAsAtomicUnit=on
  Integrator : Integrator
  I : Outport
  F : Outport  Port=2
  wires:
  Integrator/1 -> Electromagnet/1(I), I/1
  Electromagnet/1(dI_dt) -> Integrator/1
  Electromagnet/2(F) -> F/1
  V/1 -> Electromagnet/2(V)
  d/1 -> Electromagnet/3(d)

== system main_model/RMR RMA SDC MCCE/RMH2/RMR/FB Linearized EIR2/Driver ==
  "I " : Inport
  I_ref : Inport  Port=2
  Gain : Gain  Gain=K
  Saturation : Saturate
  Sum : Sum  Inputs=|+-
  V : Outport
  wires:
  Saturation/1 -> V/1
  Sum/1 -> Gain/1
  Gain/1 -> Saturation/1
  "I "/1 -> Sum/2
  I_ref/1 -> Sum/1

== system main_model/RMR RMA SDC MCCE/RMH2/RMR/FB Linearized EIR2/EIR ==
  V : Inport
  d : Inport  Port=2
  Electromagnet : MATLAB Function  TreatAsAtomicUnit=on
  Integrator : Integrator
  I : Outport
  F : Outport  Port=2
  wires:
  Integrator/1 -> Electromagnet/1(I), I/1
  Electromagnet/1(dI_dt) -> Integrator/1
  Electromagnet/2(F) -> F/1
  V/1 -> Electromagnet/2(V)
  d/1 -> Electromagnet/3(d)

== system main_model/RMR RMA SDC MCCE/RMH2/RMR/FB Linearized EIR3/Driver ==
  "I " : Inport
  I_ref : Inport  Port=2
  Gain : Gain  Gain=K
  Saturation : Saturate
  Sum : Sum  Inputs=|+-
  V : Outport
  wires:
  Saturation/1 -> V/1
  Sum/1 -> Gain/1
  Gain/1 -> Saturation/1
  "I "/1 -> Sum/2
  I_ref/1 -> Sum/1

== system main_model/RMR RMA SDC MCCE/RMH2/RMR/FB Linearized EIR3/EIR ==
  V : Inport
  d : Inport  Port=2
  Electromagnet : MATLAB Function  TreatAsAtomicUnit=on
  Integrator : Integrator
  I : Outport
  F : Outport  Port=2
  wires:
  Integrator/1 -> Electromagnet/1(I), I/1
  Electromagnet/1(dI_dt) -> Integrator/1
  Electromagnet/2(F) -> F/1
  V/1 -> Electromagnet/2(V)
  d/1 -> Electromagnet/3(d)

== system main_model/RMR RMA SDC MCCE/RMH2/RMR/FB Linearized EIR4/Driver ==
  "I " : Inport
  I_ref : Inport  Port=2
  Gain : Gain  Gain=K
  Saturation : Saturate
  Sum : Sum  Inputs=|+-
  V : Outport
  wires:
  Saturation/1 -> V/1
  Sum/1 -> Gain/1
  Gain/1 -> Saturation/1
  "I "/1 -> Sum/2
  I_ref/1 -> Sum/1

== system main_model/RMR RMA SDC MCCE/RMH2/RMR/FB Linearized EIR4/EIR ==
  V : Inport
  d : Inport  Port=2
  Electromagnet : MATLAB Function  TreatAsAtomicUnit=on
  Integrator : Integrator
  I : Outport
  F : Outport  Port=2
  wires:
  Integrator/1 -> Electromagnet/1(I), I/1
  Electromagnet/1(dI_dt) -> Integrator/1
  Electromagnet/2(F) -> F/1
  V/1 -> Electromagnet/2(V)
  d/1 -> Electromagnet/3(d)

== system main_model/RMR RMA SDC MCCE/RMH2/RMR/FB Linearized EIR5/Driver ==
  "I " : Inport
  I_ref : Inport  Port=2
  Gain : Gain  Gain=K
  Saturation : Saturate
  Sum : Sum  Inputs=|+-
  V : Outport
  wires:
  Saturation/1 -> V/1
  Sum/1 -> Gain/1
  Gain/1 -> Saturation/1
  "I "/1 -> Sum/2
  I_ref/1 -> Sum/1

== system main_model/RMR RMA SDC MCCE/RMH2/RMR/FB Linearized EIR5/EIR ==
  V : Inport
  d : Inport  Port=2
  Electromagnet : MATLAB Function  TreatAsAtomicUnit=on
  Integrator : Integrator
  I : Outport
  F : Outport  Port=2
  wires:
  Integrator/1 -> Electromagnet/1(I), I/1
  Electromagnet/1(dI_dt) -> Integrator/1
  Electromagnet/2(F) -> F/1
  V/1 -> Electromagnet/2(V)
  d/1 -> Electromagnet/3(d)

== system main_model/RMR RMA SDC MCCE/RMH2/RMR/FB Linearized EIR6/Driver ==
  "I " : Inport
  I_ref : Inport  Port=2
  Gain : Gain  Gain=K
  Saturation : Saturate
  Sum : Sum  Inputs=|+-
  V : Outport
  wires:
  Saturation/1 -> V/1
  Sum/1 -> Gain/1
  Gain/1 -> Saturation/1
  "I "/1 -> Sum/2
  I_ref/1 -> Sum/1

== system main_model/RMR RMA SDC MCCE/RMH2/RMR/FB Linearized EIR6/EIR ==
  V : Inport
  d : Inport  Port=2
  Electromagnet : MATLAB Function  TreatAsAtomicUnit=on
  Integrator : Integrator
  I : Outport
  F : Outport  Port=2
  wires:
  Integrator/1 -> Electromagnet/1(I), I/1
  Electromagnet/1(dI_dt) -> Integrator/1
  Electromagnet/2(F) -> F/1
  V/1 -> Electromagnet/2(V)
  d/1 -> Electromagnet/3(d)

== matlab function main_model/RMR RMA SDC MCCE/RMH2/MCCE/mechanism ==
  data: T input; zpp output
function zpp  = fcn(T)
%#codegen
zpp

== matlab function main_model/RMR RMA SDC MCCE/RMH1/MCCE/mechanism ==
  data: T input; zpp output
function zpp  = fcn(T)
%#codegen
zpp

== matlab function main_model/RMR RMA SDC MCCE/RMH1/MCCE/motor ==
  data: u input; y output; Ve input
function y  = fcn(u, Ve)
%#codegen
y = 0;

== matlab function main_model/RMR RMA SDC MCCE/RMH2/MCCE/motor ==
  data: u input; y output; Ve input
function y  = fcn(u, Ve)
%#codegen
y = 0;

== matlab function main_model/RMR RMA SDC MCCE/RMH2/MCCE/permanent magnet ==
  data: d input; F output
function F  = fcn(d)
%#codegen

d = 0;

== matlab function main_model/RMR RMA SDC MCCE/RMH1/MCCE/permanent magnet ==
  data: d input; F output
function F  = fcn(d)
%#codegen

d = 0;

== matlab function main_model/RMR RMA SDC MCCE/RMH1/RMA/FB Linearized EIA1/EIR/Electromagnet ==
  data: I input; V input; d input; dI_dt output; F output
function [dI_dt, F]  = fcn(I, V, d)
%#codegen

dI_dt = 0;
F = 0;

== matlab function main_model/RMR RMA SDC MCCE/RMH2/RMA/FB Linearized EIA1/EIR/Electromagnet ==
  data: I input; V input; d input; dI_dt output; F output
function [dI_dt, F]  = fcn(I, V, d)
%#codegen

dI_dt = 0;
F = 0;

== matlab function main_model/RMR RMA SDC MCCE/RMH2/RMA/FB Linearized EIA1/Force-to-current ==
  data: F_ref input; I_ref output; d input
function I_ref = fcn(F_ref, d)
%#codegen

I_ref = 0;

== matlab function main_model/RMR RMA SDC MCCE/RMH2/RMA/Force Selector ==
  data: Fx input; F1 output
function F1  = fcn(Fx)
%#codegen

F1 = 0; 
F2 = 0;
F3 = 0;
F4 = 0;
F5 = 0;
F6 = 0;

d1 = 0;
d2 = 0;
d3 = 0;
d4 = 0;
d5 = 0;
d6 = 0;

== matlab function main_model/RMR RMA SDC MCCE/RMH2/RMR/FB Linearized EIR1/EIR/Electromagnet ==
  data: I input; V input; d input; dI_dt output; F output
function [dI_dt, F]  = fcn(I, V, d)
%#codegen

dI_dt = 0;
F = 0;

== matlab function main_model/RMR RMA SDC MCCE/RMH2/RMR/FB Linearized EIR1/Force-to-current ==
  data: F_ref input; I_ref output; d input
function I_ref = fcn(F_ref, d)
%#codegen

I_ref = 0;

== matlab function main_model/RMR RMA SDC MCCE/RMH2/RMR/FB Linearized EIR2/EIR/Electromagnet ==
  data: I input; V input; d input; dI_dt output; F output
function [dI_dt, F]  = fcn(I, V, d)
%#codegen

dI_dt = 0;
F = 0;

== matlab function main_model/RMR RMA SDC MCCE/RMH2/RMR/FB Linearized EIR2/Force-to-current ==
  data: F_ref input; I_ref output; d input
function I_ref = fcn(F_ref, d)
%#codegen

I_ref = 0;

== matlab function main_model/RMR RMA SDC MCCE/RMH2/RMR/FB Linearized EIR3/EIR/Electromagnet ==
  data: I input; V input; d input; dI_dt output; F output
function [dI_dt, F]  = fcn(I, V, d)
%#codegen

dI_dt = 0;
F = 0;

== matlab function main_model/RMR RMA SDC MCCE/RMH2/RMR/FB Linearized EIR3/Force-to-current ==
  data: F_ref input; I_ref output; d input
function I_ref = fcn(F_ref, d)
%#codegen

I_ref = 0;

== matlab function main_model/RMR RMA SDC MCCE/RMH2/RMR/FB Linearized EIR4/EIR/Electromagnet ==
  data: I input; V input; d input; dI_dt output; F output
function [dI_dt, F]  = fcn(I, V, d)
%#codegen

dI_dt = 0;
F = 0;

== matlab function main_model/RMR RMA SDC MCCE/RMH2/RMR/FB Linearized EIR4/Force-to-current ==
  data: F_ref input; I_ref output; d input
function I_ref = fcn(F_ref, d)
%#codegen

I_ref = 0;

== matlab function main_model/RMR RMA SDC MCCE/RMH2/RMR/FB Linearized EIR5/EIR/Electromagnet ==
  data: I input; V input; d input; dI_dt output; F output
function [dI_dt, F]  = fcn(I, V, d)
%#codegen

dI_dt = 0;
F = 0;

== matlab function main_model/RMR RMA SDC MCCE/RMH2/RMR/FB Linearized EIR5/Force-to-current ==
  data: F_ref input; I_ref output; d input
function I_ref = fcn(F_ref, d)
%#codegen

I_ref = 0;

== matlab function main_model/RMR RMA SDC MCCE/RMH1/RMA/FB Linearized EIA1/Force-to-current ==
  data: F_ref input; I_ref output; d input
function I_ref = fcn(F_ref, d)
%#codegen

I_ref = 0;

== matlab function main_model/RMR RMA SDC MCCE/RMH1/RMA/Force Selector ==
  data: Fx input; F1 output
function F1  = fcn(Fx)
%#codegen

F1 = 0; 
F2 = 0;
F3 = 0;
F4 = 0;
F5 = 0;
F6 = 0;

d1 = 0;
d2 = 0;
d3 = 0;
d4 = 0;
d5 = 0;
d6 = 0;

== matlab function main_model/RMR RMA SDC MCCE/RMH1/RMR/FB Linearized EIR1/EIR/Electromagnet ==
  data: I input; V input; d input; dI_dt output; F output
function [dI_dt, F]  = fcn(I, V, d)
%#codegen

dI_dt = 0;
F = 0;

== matlab function main_model/RMR RMA SDC MCCE/RMH1/RMR/FB Linearized EIR1/Force-to-current ==
  data: F_ref input; I_ref output; d input
function I_ref = fcn(F_ref, d)
%#codegen

I_ref = 0;

== matlab function main_model/RMR RMA SDC MCCE/RMH1/RMR/FB Linearized EIR2/EIR/Electromagnet ==
  data: I input; V input; d input; dI_dt output; F output
function [dI_dt, F]  = fcn(I, V, d)
%#codegen

dI_dt = 0;
F = 0;

== matlab function main_model/RMR RMA SDC MCCE/RMH1/RMR/FB Linearized EIR2/Force-to-current ==
  data: F_ref input; I_ref output; d input
function I_ref = fcn(F_ref, d)
%#codegen

I_ref = 0;

== matlab function main_model/RMR RMA SDC MCCE/RMH1/RMR/FB Linearized EIR3/EIR/Electromagnet ==
  data: I input; V input; d input; dI_dt output; F output
function [dI_dt, F]  = fcn(I, V, d)
%#codegen

dI_dt = 0;
F = 0;

== matlab function main_model/RMR RMA SDC MCCE/RMH1/RMR/FB Linearized EIR3/Force-to-current ==
  data: F_ref input; I_ref output; d input
function I_ref = fcn(F_ref, d)
%#codegen

I_ref = 0;

== matlab function main_model/RMR RMA SDC MCCE/RMH1/RMR/FB Linearized EIR4/EIR/Electromagnet ==
  data: I input; V input; d input; dI_dt output; F output
function [dI_dt, F]  = fcn(I, V, d)
%#codegen

dI_dt = 0;
F = 0;

== matlab function main_model/RMR RMA SDC MCCE/RMH1/RMR/FB Linearized EIR4/Force-to-current ==
  data: F_ref input; I_ref output; d input
function I_ref = fcn(F_ref, d)
%#codegen

I_ref = 0;

== matlab function main_model/RMR RMA SDC MCCE/RMH2/RMR/FB Linearized EIR6/EIR/Electromagnet ==
  data: I input; V input; d input; dI_dt output; F output
function [dI_dt, F]  = fcn(I, V, d)
%#codegen

dI_dt = 0;
F = 0;

== matlab function main_model/RMR RMA SDC MCCE/RMH1/RMR/FB Linearized EIR5/EIR/Electromagnet ==
  data: I input; V input; d input; dI_dt output; F output
function [dI_dt, F]  = fcn(I, V, d)
%#codegen

dI_dt = 0;
F = 0;

== matlab function main_model/RMR RMA SDC MCCE/RMH1/RMR/FB Linearized EIR5/Force-to-current ==
  data: F_ref input; I_ref output; d input
function I_ref = fcn(F_ref, d)
%#codegen

I_ref = 0;

== matlab function main_model/RMR RMA SDC MCCE/RMH1/RMR/FB Linearized EIR6/EIR/Electromagnet ==
  data: I input; V input; d input; dI_dt output; F output
function [dI_dt, F]  = fcn(I, V, d)
%#codegen

dI_dt = 0;
F = 0;

== matlab function main_model/RMR RMA SDC MCCE/RMH1/RMR/FB Linearized EIR6/Force-to-current ==
  data: F_ref input; I_ref output; d input
function I_ref = fcn(F_ref, d)
%#codegen

I_ref = 0;

== matlab function main_model/RMR RMA SDC MCCE/RMH1/RMR/Force Selector ==
  data: Fy input; Fz input; dy input; F1 output; d1 output; F2 output; d2 output; F3 output; d3 output; F4 output; d4 output; F5 output; d5 output; F6 output; dz input; d6 output
function [F1, d1, F2, d2, F3, d3, F4, d4, F5, d5, F6, d6] = fcn(Fy, Fz, dy, dz)
%#codegen

F1 = 0;
F2 = 0;
F3 = 0;
F4 = 0;
F5 = 0;
F6 = 0;

d1 = 0;
d2 = 0;
d3 = 0;
d4 = 0;
d5 = 0;
d6 = 0;

== matlab function main_model/RMR RMA SDC MCCE/RMH1/RMR/Total Plane Force ==
  data: F1 input; F2 input; Fy output; Fz output; F3 input; F4 input; F5 input; F6 input
function [Fy, Fz] = fcn(F1, F2, F3, F4, F5, F6)
%#codegen
Fy = 0;
Fz = 0;

== matlab function main_model/RMR RMA SDC MCCE/RMH2/RMR/FB Linearized EIR6/Force-to-current ==
  data: F_ref input; I_ref output; d input
function I_ref = fcn(F_ref, d)
%#codegen

I_ref = 0;

== matlab function main_model/RMR RMA SDC MCCE/RMH2/RMR/Force Selector ==
  data: Fy input; Fz input; dy input; F1 output; d1 output; F2 output; d2 output; F3 output; d3 output; F4 output; d4 output; F5 output; d5 output; F6 output; dz input; d6 output
function [F1, d1, F2, d2, F3, d3, F4, d4, F5, d5, F6, d6] = fcn(Fy, Fz, dy, dz)
%#codegen

F1 = 0;
F2 = 0;
F3 = 0;
F4 = 0;
F5 = 0;
F6 = 0;

d1 = 0;
d2 = 0;
d3 = 0;
d4 = 0;
d5 = 0;
d6 = 0;

== matlab function main_model/RMR RMA SDC MCCE/RMH2/RMR/Total Plane Force ==
  data: F1 input; F2 input; Fy output; Fz output; F3 input; F4 input; F5 input; F6 input
function [Fy, Fz] = fcn(F1, F2, F3, F4, F5, F6)
%#codegen
Fy = 0;
Fz = 0;

== matlab function main_model/RMR RMA SDC MCCE/RMH2/SDC Axial/SDC Axial 1 ==
  data: d_real input; d_sense output
function d_sense  = fcn(d_real)
%#codegen
d_sense = 0;

== matlab function main_model/RMR RMA SDC MCCE/RMH2/SDC Radial/SDC Radial 1 ==
  data: d_real input; d_sense output
function d_sense  = fcn(d_real)
%#codegen
d_sense = 0;

== matlab function main_model/RMR RMA SDC MCCE/RMH2/SDC Radial/SDC Radial 2 ==
  data: d_real input; d_sense output
function d_sense  = fcn(d_real)
%#codegen
d_sense = 0;

== matlab function main_model/RMR RMA SDC MCCE/RMH2/SDC Radial/SDC Radial 3 ==
  data: d_real input; d_sense output
function d_sense  = fcn(d_real)
%#codegen
d_sense = 0;

== matlab function main_model/RMR RMA SDC MCCE/RMH2/SDC Radial/Sensor Selector ==
  data: dy input; d1 output; d2 output; d3 output; dz input
function [d1,d2,d3] = fcn(dy,dz)
%#codegen
d1 = 0;
d2 = 0;
d3 = 0;

== matlab function main_model/RMR RMA SDC MCCE/RMH1/SDC Axial/SDC Axial 1 ==
  data: d_real input; d_sense output
function d_sense  = fcn(d_real)
%#codegen
d_sense = 0;

== matlab function main_model/RMR RMA SDC MCCE/RMH1/SDC Radial/SDC Radial 1 ==
  data: d_real input; d_sense output
function d_sense  = fcn(d_real)
%#codegen
d_sense = 0;

== matlab function main_model/RMR RMA SDC MCCE/RMH1/SDC Radial/SDC Radial 2 ==
  data: d_real input; d_sense output
function d_sense  = fcn(d_real)
%#codegen
d_sense = 0;

== matlab function main_model/RMR RMA SDC MCCE/RMH1/SDC Radial/SDC Radial 3 ==
  data: d_real input; d_sense output
function d_sense  = fcn(d_real)
%#codegen
d_sense = 0;

== matlab function main_model/RMR RMA SDC MCCE/RMH1/SDC Radial/Sensor Selector ==
  data: dy input; d1 output; d2 output; d3 output; dz input
function [d1,d2,d3] = fcn(dy,dz)
%#codegen
d1 = 0;
d2 = 0;
d3 = 0;

== matlab function main_model/RMR RMA SDC MCCE/RMH2/SDC Radial/position calc ==
  data: d1 input; d2 input; dy_sense output; dz_sense output; d3 input
function [dy_sense, dz_sense] = fcn(d1,d2,d3)
%#codegen
dy_sense = 0;
dz_sense = 0;

== matlab function main_model/RMR RMA SDC MCCE/RMH1/SDC Radial/position calc ==
  data: d1 input; d2 input; dy_sense output; dz_sense output; d3 input
function [dy_sense, dz_sense] = fcn(d1,d2,d3)
%#codegen
dy_sense = 0;
dz_sense = 0;

== matlab function main_model/RMR RMA SDC MCCE/MATLAB Function ==
  data: x0 input; SDC1_dx output; y0 input; z0 input; phi input; theta input; RMA1_dx output; RMR1_dy output; RMR1_dz output; SDC1_dy output; SDC1_dz output; MCCE1_dz output; SDC2_dx output; RMA2_dx output; RMR2_dy output; RMR2_dz output; SDC2_dy output; SDC2_dz output; MCCE2_dz output
function [SDC1_dx, RMA1_dx, RMR1_dy, RMR1_dz, SDC1_dy, SDC1_dz, MCCE1_dz, SDC2_dx, RMA2_dx, RMR2_dy, RMR2_dz, SDC2_dy, SDC2_dz, MCCE2_dz] = fcn(x0,y0,z0,phi,theta)
%#codegen
SDC1_dx = 0;
RMA1_dx = 0;
RMR1_dy = 0;
RMR1_dz = 0;
SDC1_dy = 0;
SDC1_dz = 0;
MCCE1_dz = 0;

SDC2_dx = 0;
RMA2_dx = 0;
RMR2_dy = 0;
RMR2_dz = 0;
SDC2_dy = 0;
SDC2_dz = 0;
MCCE2_dz = 0;
